simulink model "Projeto_Final_versao_1_M21"  (R2021a)
settings: Solver=VariableStepAuto  StartTime=0  StopTime=144  FixedStep=0.1  RelTol=1e-3
model workspace (MAT data in the model file):
  N_P0 = 3
  variavelteste = 0
libraries: spsACVoltageSourceLib x1, spsCurrentMeasurementLib x1, spsSeriesRLCBranchLib x1, autolibsharedmappedengines x1, spspowerguiLib x1
(part 1 of 4)
settings Model: EnablePacing=on  Creator=Henrique  LastModifiedBy=Desktop

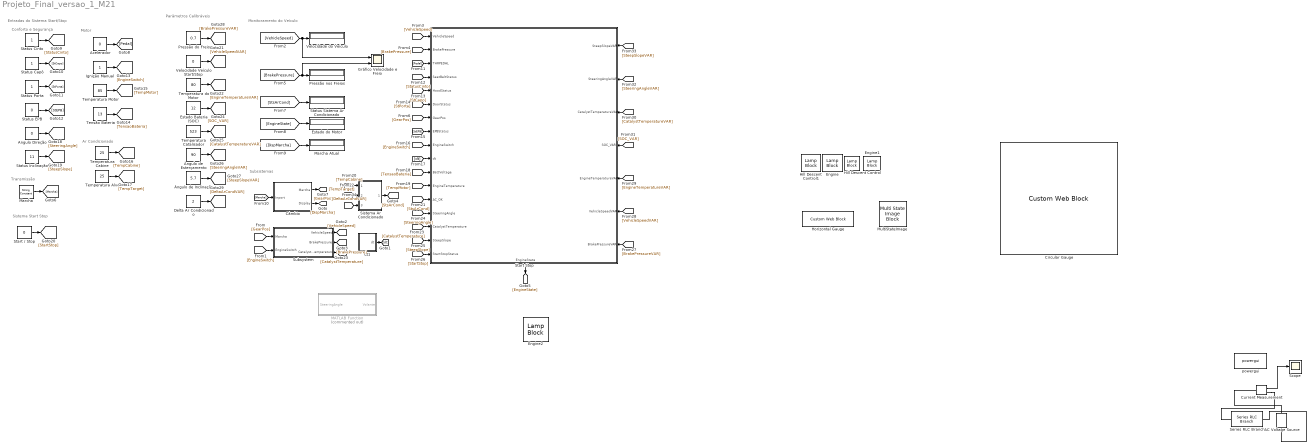
== system Projeto_Final_versao_1_M21 ==
  note: Sistema Start Stop
  note: Transmissão
  note: Motor
  note: Conforto e Segurança
  note: Ar Condicionado
  note: Entradas do Sistema Start/Stop
  note: Subsistemas
  note: Monitoramento do Veículo
  note: Parâmetros Calibráveis
  AC Voltage Source : spsACVoltageSourceLib/AC Voltage Source  Amplitude=100  Phase=0  Frequency=60  SampleTime=0  Measurements=None  BusType=swing  Pref=10e3  Qref=0  Qmin=-inf  Qmax=+inf
  Acelerador : Constant  Value=0
  Angulo Direção : Constant  Value=0
  Circular Gauge : CustomWebBlock  LabelPosition=Hide  ShowInitialText=on  Configuration="{\"components\":[{\"name\":\"CircularScaleComponent\",\"settings\":{\"bounds\":{\"max\":100,\"min\":0,\"tickInterval\":\"auto\"},\"direction\":\"cw\",\"flipLimits\":0,\"innerRadius\":0.75,\"internalTickHeightScaleFactor\":1,\"labelColor\":[255,255,200],\"labelFont\":{\"font\":\"Arial\",\"fontSize\":12},\"labelTransparency\":1,\"minorTickHeightScaleFactor\":0.2,\"needleImage\":{\"size\":[200,50],\"src\":\"data:image\\/svg+xml;base64,PD94bWwgdmVyc2lvbj0iMS4wIiBlbmNvZGluZz0idXRmLTgiPz4KPCEtLSBHZW5lcmF0b3I6IEFkb2JlIElsbHVzdHJhdG9yIDI0LjEuMiwgU1ZHIEV4cG9ydCBQbHVnLUluIC4gU1ZHIFZlcnNpb246IDYuMDAgQnVpbGQgMCkgIC0tPgo8c3ZnIHZlcnNpb249IjEuMSIgaWQ9IkxheWVyXzEiIHhtbG5zPSJodHRwOi8vd3d3LnczLm9yZy8yMDAwL3N2ZyIgeG1sbnM6eGxpbms9Imh0dHA6Ly93d3cudzMub3JnLzE5OTkveGxpbmsiIHg9IjBweCIgeT0iMHB4IgoJIHZpZXdCb3g9IjAgMCAyMDAgNTAiIHN0eWxlPSJlbmFibGUtYmFja2dyb3VuZDpuZXcgMCAwIDIwMCA1MDsiIHhtbDpzcGFjZT0icHJlc2VydmUiPgo8c3R5bGUgdHlwZT0idGV4dC9jc3MiPgoJLnN0MHtmaWxsOiNFQzIxMjc7fQo8L3N0eWxlPgo8cGF0aCBjbGFzcz0ic3QwIiBkPSJNMTYyLjgsMTMuN0MxNjksNC40LDE4MS43LDEuOSwxOTEsOC4xczExLjgsMTguOSw1LjYsMjguMnMtMTguOSwxMS44LTI4LjIsNS42bDAsMAoJQzE1OS4xLDM1LjYsMTU2LjYsMjMsMTYyLjgsMTMuN0wxNjIuOCwxMy43eiBNMTY1LjgsMTUuOGMtNS4xLDcuNi0zLjEsMTcuOSw0LjYsMjNjNy42LDUuMSwxNy45LDMuMSwyMy00LjYKCWM1LjEtNy42LDMuMS0xNy45LTQuNi0yM2wwLDBDMTgxLjIsNi4yLDE3MC45LDguMiwxNjUuOCwxNS44eiIvPgo8cGF0aCBjbGFzcz0ic3QwIiBkPSJNMC40LDI1Ljl2LTMuM2wxNTktMi41Yy0wLjcsMi42LTAuNyw1LjIsMCw3LjhMMC40LDI1Ljl6Ii8+CjxjaXJjbGUgY2xhc3M9InN0MCIgY3g9IjE3OS42IiBjeT0iMjQiIHI9IjAuNyIvPgo8L3N2Zz4K\"},\"needleOffset\":[0.18464878250906522,0],\"needleOrientation\":-45,\"needleRotation\":180,\"needleSize\":{\"height\":0.11741692305346914,\"width\":0.46108337545091255},\"outerRadius\":0.9,\"position\":[0.06486742424242424,0.05627705627705628,0.8917748917748918,0.8787878787878788],\"scaleAngle\":270,\"scaleAngleOffset\":135,\"scaleColors\":[],\"scaleColorsSize\":0.2,\"scalePosition\":[0,0,1,1],\"showLabels\":1,\"showMinorTicks\":1,\"showSpanLine\":1,\"showTicks\":1,\"tickColor\":[252,252,197],\"tickTransparency\":1,\"valueBarColor\":[0,114,189],\"valueBarPosition\":[0,0,1,1],\"valueBarSize\":0.2,\"valueBarTransparency\":1}},{\"name\":\"BackgroundImageComponent\",\"settings\":{\"image\":{\"size\":[500,500],\"src\":\"data:image\\/svg+xml;base64,PD94bWwgdmVyc2lvbj0iMS4wIiBlbmNvZGluZz0iVVRGLTgiIHN0YW5kYWxvbmU9Im5vIj8+CjxzdmcKICAgeG1sbnM6ZGM9Imh0dHA6Ly9wdXJsLm9yZy9kYy9lbGVtZW50cy8xLjEvIgogICB4bWxuczpjYz0iaHR0cDovL2NyZWF0aXZlY29tbW9ucy5vcmcvbnMjIgogICB4bWxuczpyZGY9Imh0dHA6Ly93d3cudzMub3JnLzE5OTkvMDIvMjItcmRmLXN5bnRheC1ucyMiCiAgIHhtbG5zOnN2Zz0iaHR0cDovL3d3dy53My5vcmcvMjAwMC9zdmciCiAgIHhtbG5zPSJodHRwOi8vd3d3LnczLm9yZy8yMDAwL3N2ZyIKICAgeG1sbnM6 ...(+9964 chars)\"},\"position\":[0,0,1,1],\"scaleMode\":\"0\"}},{\"name\":\"ForegroundImageComponent\",\"settings\":{\"image\":{\"size\":[0,0],\"src\":\"default\",\"srcOrientation\":[]},\"isForeground\":1,\"position\":[0,0,1,1],\"scaleMode\":\"0\"}}],\"settings\":{\"BindingType\":\"signal\",\"aspectRatio\":1.032258064516129,\"backgroundColor\":[0,0,0,\"1\"],\"backgroundOffset\":0.14,\"backgroundOpacity\":1,\"direction\":\"cw\",\"fixedAspectRatio\":\"on\",\"flipLimits\":0,\"orientation\":\"horizontal\",\"showBackgroundColor\":false,\"value\":0},\"type\":\"CircularGauge\"}"
  Current Measurement : spsCurrentMeasurementLib/Current Measurement  PhasorSimulation=off  OutputType=Complex  PSBequivalent=0
  Câmbio : Subsystem
  Delta Ar Condicionado : Constant  Value=2
  Engine : LampBlock  LabelPosition=Hide  Icon=Engine
  Engine1 : LampBlock  LabelPosition=Hide  Icon=Custom  CustomIcon=data:image/svg+xml;base64,PD94bWwgdmVyc2lvbj0iMS4wIiBlbmNvZGluZz0iaXNvLTg4NTktMSI/Pg0KPCEtLSBVcGxvYWRlZCB0bzogU1ZHIFJlcG8sIHd3dy5zdmdyZXBvLmNvbSwgR2VuZXJhdG9yOiBTVkcgUmVwbyBNaXhlciBUb29scyAtLT4NCjxzdmcgZmlsbD0iIzAwMDAwMCIgaGVpZ2h0PSI4MDBweCIgd2lkdGg9IjgwMHB4IiB2ZXJzaW9uPSIxLjEiIGlkPSJMYXllcl8xIiB4bWxucz0iaHR0cDovL3d3dy53My5vcmcvMjAwMC9zdmciIHhtbG5zOnhsaW5rPSJodHRwOi8vd3d3LnczLm9yZy8xOTk5L3hsaW5rIiANCgkgdmlld0JveD0iMCAwIDUx ...(+2036 chars)
  Engine2 : LampBlock  LabelPosition=Hide  Icon=Custom  CustomIcon=data:image/svg+xml;base64,PD94bWwgdmVyc2lvbj0iMS4wIiBlbmNvZGluZz0iaXNvLTg4NTktMSI/Pg0KPCEtLSBVcGxvYWRlZCB0bzogU1ZHIFJlcG8sIHd3dy5zdmdyZXBvLmNvbSwgR2VuZXJhdG9yOiBTVkcgUmVwbyBNaXhlciBUb29scyAtLT4NCjxzdmcgZmlsbD0iIzAwMDAwMCIgaGVpZ2h0PSI4MDBweCIgd2lkdGg9IjgwMHB4IiB2ZXJzaW9uPSIxLjEiIGlkPSJDYXBhXzEiIHhtbG5zPSJodHRwOi8vd3d3LnczLm9yZy8yMDAwL3N2ZyIgeG1sbnM6eGxpbms9Imh0dHA6Ly93d3cudzMub3JnLzE5OTkveGxpbmsiIA0KCSB2aWV3Qm94PSIwIDAgNjEy ...(+1612 chars)
  Estado Bateria (SOC) : Constant  Value=12
  Estado do Motor : Display
  Gráfico Velocidade e Freio : Scope  NumInputPorts=2
  Hill Descent Control : LampBlock  LabelPosition=Hide  Icon=Custom  CustomIcon=data:image/svg+xml;base64,PD94bWwgdmVyc2lvbj0iMS4wIiBlbmNvZGluZz0iaXNvLTg4NTktMSI/Pg0KPCEtLSBVcGxvYWRlZCB0bzogU1ZHIFJlcG8sIHd3dy5zdmdyZXBvLmNvbSwgR2VuZXJhdG9yOiBTVkcgUmVwbyBNaXhlciBUb29scyAtLT4NCjxzdmcgZmlsbD0iIzAwMDAwMCIgdmVyc2lvbj0iMS4xIiBpZD0iTGF5ZXJfMSIgeG1sbnM9Imh0dHA6Ly93d3cudzMub3JnLzIwMDAvc3ZnIiB4bWxuczp4bGluaz0iaHR0cDovL3d3dy53My5vcmcvMTk5OS94bGluayIgDQoJIHZpZXdCb3g9IjAgMCA1MTIgNTEyIiB4bWw6c3BhY2U9InByZXNlcnZlIj4NCjxnPg0KCTxnPg0KCQk8cGF0aCBkPSJNNTA2LjU4Myw5Ljg0N0M1MDEuNzI3LDMuNjM1LDQ5NC4yODYsMCw0ODYuNDAyLDBoLTI1NmMtNi43OTMsMC0xMy4zMDMsMi42OTctMTguMDk5LDcuNTAxbC0yMDQuOCwyMDQuOA0KCQkJYy00LjgwNCw0Ljc5Ni03LjUwMSwxMS4zMDctNy41MDEsMTguMDk5djI1NmMwLDE0LjE0LDExLjQ2LDI1LjYsMjUuNiwyNS42aDQwOS42YzE0LjE0LDAsMjUuNi0xMS40NiwyNS42LTI1LjZWMjMzLjU0OQ0KCQkJbDUwLjQzMi0yMDEuNzQ1QzUxMy4xNDUsMjQuMTU4LDUxMS40MywxNi4wNiw1MDYuNTgzLDkuODQ3eiBNNDM1LjIwMiw0ODYuNGgtNDA5LjZWMjU2aDQwOS42VjQ4Ni40eiBNNDM1LjIwMiwyMzAuNGgtNDA5LjYNCgkJCWwyMDQuOC0yMDQuOGgyNTZMNDM1LjIwMiwyMzAuNHoiLz4NCgk8L2c+DQo8L2c+DQo8Zz4NCgk8Zz4NCgkJPHJlY3QgeD0iMzMyLjgwMiIgeT0iMjgxLjYiIHdpZHRoPSI3Ni44IiBoZWlnaHQ9IjI1LjYiLz4NCgk8L2c+DQo8L2c+DQo8L3N2Zz4=
  Hill Descent Control1 : LampBlock  LabelPosition=Hide  Icon=Custom  CustomIcon=data:image/svg+xml;base64,PHN2ZyB4bWxucz0iaHR0cDovL3d3dy53My5vcmcvMjAwMC9zdmciIHdpZHRoPSIxMDI0IiBoZWlnaHQ9IjEwMjQiIHZpZXdCb3g9IjAgMCAxMDI0IDEwMjQiPgogIDxwYXRoIGQ9Ik0gNzM2IDIwOCBMIDczNSAyMDkgTCA3MzIgMjA5IEwgNzMxIDIxMCBMIDczMCAyMTAgTCA3MjggMjEyIEwgNzI3IDIxMiBMIDcyMyAyMTYgTCA3MjMgMjE3IEwgNjg5IDI1MSBMIDY4OSAyNTIgTCA2ODggMjUzIEwgNjg3IDI1MyBMIDY4MiAyNTggTCA2ODIgMjU5IEwgNjgwIDI2MSBMIDY3OSAyNjEgTCA2NzcgMjYzIEwgNjc3IDI2NCBMIDYwOSAz ...(+20488 chars)
  Horizontal Gauge : CustomWebBlock  LabelPosition=Hide  ShowInitialText=on  Configuration="{\"components\":[{\"name\":\"LinearScaleComponent\",\"settings\":{\"bounds\":{\"max\":1,\"min\":0,\"tickInterval\":\"auto\"},\"internalTickHeightScaleFactor\":0.5,\"labelColor\":[255,255,200],\"labelFont\":{\"font\":\"Arial\",\"fontSize\":12},\"labelTransparency\":1,\"needleImage\":{\"size\":[21,75],\"src\":\"data:image\\/svg+xml;base64,PHN2ZyB4bWxucz0iaHR0cDovL3d3dy53My5vcmcvMjAwMC9zdmciIHhtbG5zOnhsaW5rPSJodHRwOi8vd3d3LnczLm9yZy8xOTk5L3hsaW5rIiB2aWV3Qm94PSIwIDAgMjEgNzUiPjxkZWZzPjxzdHlsZT4uY2xzLTF7ZmlsbDpub25lO30uY2xzLTJ7aXNvbGF0aW9uOmlzb2xhdGU7fS5jbHMtM3tjbGlwLXBhdGg6dXJsKCNjbGlwLXBhdGgpO30uY2xzLTR7b3BhY2l0eTowLjM7bWl4LWJsZW5kLW1vZGU6bXVsdGlwbHk7fS5jbHMtNXtmaWxsOiNlYjI2Mjk7fTwvc3R5bGU+PGNsaXBQYXRoIGlkPSJjbGlwLXBhdGgiIHRyYW5zZm9y ...(+1928 chars)\",\"srcOrientation\":\"horizontal\"},\"needleOffset\":[0,0.01094391244870041],\"needleSize\":{\"height\":0.7589285714285714,\"width\":0.11960078534031414},\"position\":[0.06986607142857143,0.01995798319327731,0.9641544117647058,0.8],\"scaleColors\":[],\"scaleColorsSize\":0.2,\"showLabels\":1,\"showMinorTicks\":0,\"showSpanLine\":1,\"showTicks\":1,\"tickColor\":[252,252,197],\"tickTransparency\":1,\"valueBarColor\":[23,89,176],\"valueBarOffset\":0,\"valueBarSize\":0.23,\"valueBarTransparency\":1}},{\"name\":\"BackgroundImageComponent\",\"settings\":{\"image\":{\"size\":[380,101],\"src\":\"data:image\\/svg+xml;base64,PHN2ZyB4bWxucz0iaHR0cDovL3d3dy53My5vcmcvMjAwMC9zdmciIHZpZXdCb3g9IjAgMCAzODAgMTAxIj48ZGVmcz48c3R5bGU+LmNscy0xe2ZpbGw6IzAwMmI0Mjt9LmNscy0ye2ZpbGw6IzQyNzA4Mjt9LmNscy0ze2ZpbGw6IzdjYTBiMjt9PC9zdHlsZT48L2RlZnM+PHRpdGxlPmhvcml6b250YWxfZ2F1Z2VfIGJhY2tncm91bmQ8L3RpdGxlPjxnIGlkPSJMYXllcl8yIiBkYXRhLW5hbWU9IkxheWVyIDIiPjxnIGlkPSJMYXllcl8xLTIiIGRhdGEtbmFtZT0iTGF5ZXIgMSI+PHJlY3QgY2xhc3M9ImNscy0xIiB4PSIxMSIgeT0iMTEiIHdpZHRoPSIzNTgiIGhlaWdodD0iNzkiLz48cGF0aCBjbGFzcz0iY2xzLTIiIGQ9Ik04LDhWOTNIMzcyVjhaTTM2OSw5MEgxMVYxMUgzNjlaIi8+PHBhdGggY2xhc3M9ImNscy0zIiBkPSJNMCwwVjEwMUgzODBWMFpNMzcyLDkzSDhWOEgzNzJaIi8+PC9nPjwvZz48L3N2Zz4=\",\"srcOrientation\":\"horizontal\"},\"position\":[0,0,1,1],\"scaleMode\":\"0\"}},{\"name\":\"ForegroundImageComponent\",\"settings\":{\"image\":{\"size\":[0,0],\"src\":\"default\",\"srcOrientation\":[]},\"isForeground\":1,\"position\":[0,0,1,1],\"scaleMode\":\"0\"}}],\"settings\":{\"BindingType\":\"signal\",\"backgroundColor\":[0,0,0,\"1\"],\"backgroundOffset\":0,\"backgroundOpacity\":1,\"fixedAspectRatio\":\"on\",\"orientation\":\"horizontal\",\"showBackgroundColor\":false,\"value\":0},\"type\":\"LinearGauge\"}"
  Ignição Manual : Constant
  MATLAB Function : MATLAB Function  Commented=on  TreatAsAtomicUnit=on
  Marcha : StringConstant  String="\"D\""
  Marcha Atual : Display
  MultiStateImage : MultiStateImageBlock  LabelPosition=Hide
  Pressão do Freio : Constant  Value=0.7
  Pressão nos Freios : Display
  Scope : Scope
  Series RLC Branch : spsSeriesRLCBranchLib/Series RLC Branch  LConnTagsString=__new0  RConnTagsString=__new0  BranchType=RLC  Resistance=1  Inductance=1e-3  SetiL0=off  InitialCurrent=0  Capacitance=1e-6  Setx0=off  InitialVoltage=0  Measurements=None
  Sistema Ar Condicionado : Subsystem
  Start / Stop : Constant  Value=0
  Start Stop : Subsystem
      settings: PortSchema="{\"entries\":[{\"content\":{\"sides\":[{\"content\":{\"connectorIds\":[\"In1\",\"In2\",\"In3\",\"In4\",\"In5\",\"In6\",\"In7\",\"In8\",\"In9\",\"In10\",\"In11\",\"In12\",\"In13\",\"In14\",\"In15\",\"In16\",\"In17\"]},\"type\":\"ConnectorPlacement.EquallySpacedRectSide\",\"uuid\":\"cae27aae-2f0f-495d-b5de-17320b8abd8f\"},{\"content\":{\"connectorIds\":[\"In18\",\"In19\",\"In20\",\"In21\",\"In22\",\"In23\",\"In24\"],\"side\":\"RIGHT\"},\"type\":\"ConnectorPlacement.EquallySpacedRectSide\",\"uuid\":\"8e8233cc-2459-4a11-817a-071854540998\"},{\"content\":{\"connectorIds\":[],\"side\":\"TOP\"},\"type\":\"ConnectorPlacement.EquallySpacedRectSide\",\"uuid\":\"41c669d9-b680-4e51-b1b6-d6f2b3952c85\"},{\"content\":{\"connectorIds\":[\"Out1\"],\"side\":\"BOTTOM\"},\"type\":\"ConnectorPlacement.EquallySpacedRectSide\",\"uuid\":\"afe65350-4104-4111-ba67-f67e88854dc7\"}]},\"type\":\"ConnectorPlacement.EquallySpacedConnector\",\"uuid\":\"9a6ef2d3-242d-431b-b81f-5ad437d41931\"}],\"packageUris\":[\"http://schema.mathworks.com/mf0/Connector/R2020b\"],\"version\":\"1.0\"}"
  Status Capô : Constant
  Status Cinto : Constant
  Status EPB : Constant  Value=0
  Status Inclinação : Constant  Value=11
  Status Porta : Constant
  Status Sistema Ar Condicionado : Display
  Subsystem : Subsystem
  Temperatura Alvo : Constant  Value=25
  Temperatura Cabine : Constant  Value=25
  Temperatura Catalisador : Constant  Value=523
  Temperatura Motor : Constant  Value=85
  Temperatura do Motor : Constant  Value=80
  Tensão Bateria : Constant  Value=13
  Velocidade Veículo Start/Stop : Constant  Value=0
  Velocidade do Veículo : Display
  dt1 : Subsystem
  powergui : spspowerguiLib/powergui  Priority=1  SimulationMode=Continuous  SampleTime=50e-6  frequency=60  Iterations=50  frequencyindice=60  Pbase=100e6  ErrMax=1e-4  UnitsV=kV  UnitsW=MW  buscounter=0  FunctionMessages=off  echomessages=off  EnableUseOfTLC=off  CurrentSourceSwitches=off  DisableSnubberDevices=off  DisableRonSwitches=off  DisableVfSwitches=off  DisplayEquations=off  AutomaticDiscreteSolvers=off  SolverType=Tustin/Backward Euler (TBE)  Interpol=off  ExternalGateDelay=off  methode=off  Ts=100  x0status=blocks  SPID=on  SwTol=0  HookPort=off  NonlinearTolerance=1e-4  nMaxIteration=100  ContinueOnMaxIteration=off  RestoreLinks=warning  ResistiveCurrentMeasurement=off  Frange=[0:2:500]  Ylog=off  Xlog=on  ShowGrid=off  save=off  variable=ZData  structure=0  ZoomFFT=off  StartTime=0.0  cycles=1  DisplayStyle=1  fundamental=60  FreqAxis=off  MaxFrequency=1000  frequencyindicesteady=1  RmsSteady=1  display=off
  Ângulo de Esterçamento : Constant  Value=90
  Ângulo de Inclinação : Constant  Value=5.7
  wires:
  Current Measurement/1 -> Scope/1
  [dt] -> Start Stop/10(dt)
  Start Stop/1(EngineState) -> [EngineState]
  Sistema Ar Condicionado/1(AC_OK) -> [StsArCond]
  [VehicleSpeed] -> Start Stop/1(VehicleSpeed)
  [BrakePressure] -> Start Stop/2(BrakePressure)
  [VehicleSpeed] -> Gráfico Velocidade e Freio/1, Velocidade do Veículo/1
  [BrakePressure] -> Gráfico Velocidade e Freio/2, Pressão nos Freios/1
  [StsArCond] -> Status Sistema Ar Condicionado/1
  [EngineState] -> Estado do Motor/1
  [DispMarcha] -> Marcha Atual/1
  Marcha/1 -> [Marcha]
  [Marcha] -> Câmbio/1(Inport)
  Câmbio/1(Marcha) -> [GearPos]
  Câmbio/2(Display) -> [DispMarcha]
  [GearPos] -> Start Stop/7(GearPos)
  Acelerador/1 -> [Pedal]
  Status Cinto/1 -> [StatusCinto]
  Status Capô/1 -> [StCapo]
  Status Porta/1 -> [StPorta]
  Status EPB/1 -> [StEPB]
  Ignição Manual/1 -> [EngineSwitch]
  [Pedal] -> Start Stop/3(THRPEDAL)
  [StatusCinto] -> Start Stop/4(SeatBeltStatus)
  [StCapo] -> Start Stop/5(HoodStatus)
  [StPorta] -> Start Stop/6(DoorStatus)
  [StEPB] -> Start Stop/8(EPBStatus)
  [EngineSwitch] -> Start Stop/9(EngineSwitch)
  dt1/1(dt) -> [dt]
  Tensão Bateria/1 -> [TensaoBateria]
  [TensaoBateria] -> Start Stop/11(BattVoltage)
  [TempMotor] -> Start Stop/12(EngineTemperature)
  Temperatura Motor/1 -> [TempMotor]
  [StsArCond] -> Start Stop/13(AC_OK)
  [GearPos] -> Subsystem/1(Marcha)
  [EngineSwitch] -> Subsystem/2(EngineSwitch)
  Subsystem/1(VehicleSpeed) -> [VehicleSpeed]
  Subsystem/2(BrakePressure) -> [BrakePressure]
  Temperatura Alvo/1 -> [TempTarget]
  Temperatura Cabine/1 -> [TempCabine]
  [TempCabine] -> Sistema Ar Condicionado/1(CabinTemperature)
  [TempTarget] -> Sistema Ar Condicionado/2(TargetTemperature)
  [CatalystTemperature] -> Start Stop/15(CatalystTemperature)
  Angulo Direção/1 -> [SteeringAngle]
  [SteeringAngle] -> Start Stop/14(SteeringAngle)
  Status Inclinação/1 -> [SteepSlope]
  [SteepSlope] -> Start Stop/16(SteepSlope)
  Subsystem/3(CatalystTemperature) -> [CatalystTemperature]
  [StartStop] -> Start Stop/17(StartStopStatus)
  Start / Stop/1 -> [StartStop]
  Pressão do Freio/1 -> [BrakePressureVAR]
  Velocidade Veículo Start/Stop/1 -> [VehicleSpeedVAR]
  Temperatura do Motor/1 -> [EngineTemperatureVAR]
  Estado Bateria (SOC)/1 -> [SOC_VAR]
  Temperatura Catalisador/1 -> [CatalystTemperatureVAR]
  Ângulo de Esterçamento/1 -> [SteeringAngleVAR]
  Ângulo de Inclinação/1 -> [SteepSlopeVAR]
  Delta Ar Condicionado/1 -> [DeltaArCondVAR]
  [SteepSlopeVAR] -> Start Stop/18(SteepSlopeVAR)
  [SteeringAngleVAR] -> Start Stop/19(SteeringAngleVAR)
  [CatalystTemperatureVAR] -> Start Stop/20(CatalystTemperatureVAR)
  [SOC_VAR] -> Start Stop/21(SOC_VAR)
  [EngineTemperatureVAR] -> Start Stop/22(EngineTemperatureVAR)
  [VehicleSpeedVAR] -> Start Stop/23(VehicleSpeedVAR)
  [BrakePressureVAR] -> Start Stop/24(BrakePressureVAR)
  [DeltaArCondVAR] -> Sistema Ar Condicionado/3(DeltaArCondVAR)
  connections:
  AC Voltage Source/LConn1 -- Series RLC Branch/RConn1
  AC Voltage Source/RConn1 -- Current Measurement/LConn1
  Current Measurement/RConn1 -- Series RLC Branch/LConn1
